simulink model "gm_HDL_pfc_gold_fi_og_vnl"  (R2024b)
settings: Solver=FixedStepDiscrete  StartTime=0.0  StopTime=.2  RelTol=1e-3
InitFcn:
  | fidelity_pfc_vals;
  | nbits=(2^12)-2;
  | load('C:\Users\Angel\Desktop\hil\pfc3ph\matlab\sim\sschdl\pfc_desktop\stateSpaceParameters.mat');
undefined symbols (not defined in the file or in its folder): a, b, c, DiscIntNeverNeededParam, fsw, Gs, s, stateSpaceParameters_1, t_ss, tsw
libraries: simulink x47, hdlmdlgenlib x24, hdlsllib x10, mcbcontrolslib x5, dspsrcs4 x3, slpidlib x2, hdlssclib x2, spsSVPWMGenerator2LevelLib x1, spsPLL3phLib x1, fillib x1
(part 3 of 5)

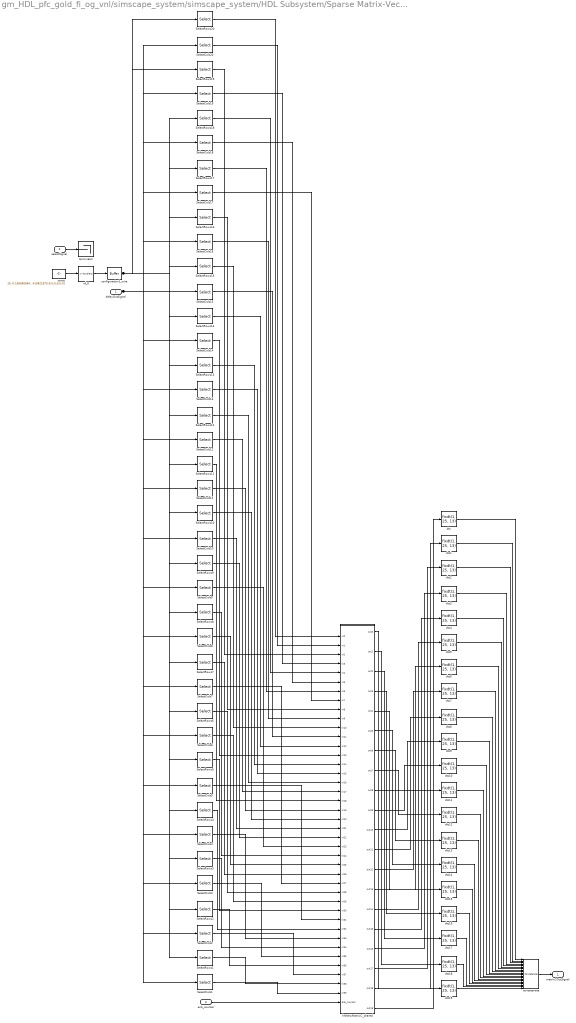
== system gm_HDL_pfc_gold_fi_og_vnl/simscape_system/simscape_system/HDL Subsystem/Sparse Matrix-Vector Product2 ==
  delayOutSignal : Inport  OutDataTypeStr=fixdt(1, 25, 13)  PortDimensions=[7]  SampleTime=1.38600138600139e-08
  selectSignal : Inport  Port=2  OutDataTypeStr=boolean  SampleTime=1.38600138600139e-08
  enb_counter : Inport  Port=3  OutDataTypeStr=fixdt(0, 6, 0)  SampleTime=1.38600138600139e-08
  SelectCols{1..20} (20 alike) : Selector  InputPortWidth=7  IndexOptions=Index vector (dialog)  Indices=double([1 2 3 4 5 6 7])  OutputSizes=double(1)
  SelectRows1 : Selector  InputPortWidth=140  IndexOptions=Index vector (dialog)  Indices=double([1 21 41 61 81 101 121])  OutputSizes=double(1)
  SelectRows10 : Selector  InputPortWidth=140  IndexOptions=Index vector (dialog)  Indices=double([10 30 50 70 90 110 130])  OutputSizes=double(1)
  SelectRows11 : Selector  InputPortWidth=140  IndexOptions=Index vector (dialog)  Indices=double([11 31 51 71 91 111 131])  OutputSizes=double(1)
  SelectRows12 : Selector  InputPortWidth=140  IndexOptions=Index vector (dialog)  Indices=double([12 32 52 72 92 112 132])  OutputSizes=double(1)
  SelectRows13 : Selector  InputPortWidth=140  IndexOptions=Index vector (dialog)  Indices=double([13 33 53 73 93 113 133])  OutputSizes=double(1)
  SelectRows14 : Selector  InputPortWidth=140  IndexOptions=Index vector (dialog)  Indices=double([14 34 54 74 94 114 134])  OutputSizes=double(1)
  SelectRows15 : Selector  InputPortWidth=140  IndexOptions=Index vector (dialog)  Indices=double([15 35 55 75 95 115 135])  OutputSizes=double(1)
  SelectRows16 : Selector  InputPortWidth=140  IndexOptions=Index vector (dialog)  Indices=double([16 36 56 76 96 116 136])  OutputSizes=double(1)
  SelectRows17 : Selector  InputPortWidth=140  IndexOptions=Index vector (dialog)  Indices=double([17 37 57 77 97 117 137])  OutputSizes=double(1)
  SelectRows18 : Selector  InputPortWidth=140  IndexOptions=Index vector (dialog)  Indices=double([18 38 58 78 98 118 138])  OutputSizes=double(1)
  SelectRows19 : Selector  InputPortWidth=140  IndexOptions=Index vector (dialog)  Indices=double([19 39 59 79 99 119 139])  OutputSizes=double(1)
  SelectRows2 : Selector  InputPortWidth=140  IndexOptions=Index vector (dialog)  Indices=double([2 22 42 62 82 102 122])  OutputSizes=double(1)
  SelectRows20 : Selector  InputPortWidth=140  IndexOptions=Index vector (dialog)  Indices=double([20 40 60 80 100 120 140])  OutputSizes=double(1)
  SelectRows3 : Selector  InputPortWidth=140  IndexOptions=Index vector (dialog)  Indices=double([3 23 43 63 83 103 123])  OutputSizes=double(1)
  SelectRows4 : Selector  InputPortWidth=140  IndexOptions=Index vector (dialog)  Indices=double([4 24 44 64 84 104 124])  OutputSizes=double(1)
  SelectRows5 : Selector  InputPortWidth=140  IndexOptions=Index vector (dialog)  Indices=double([5 25 45 65 85 105 125])  OutputSizes=double(1)
  SelectRows6 : Selector  InputPortWidth=140  IndexOptions=Index vector (dialog)  Indices=double([6 26 46 66 86 106 126])  OutputSizes=double(1)
  SelectRows7 : Selector  InputPortWidth=140  IndexOptions=Index vector (dialog)  Indices=double([7 27 47 67 87 107 127])  OutputSizes=double(1)
  SelectRows8 : Selector  InputPortWidth=140  IndexOptions=Index vector (dialog)  Indices=double([8 28 48 68 88 108 128])  OutputSizes=double(1)
  SelectRows9 : Selector  InputPortWidth=140  IndexOptions=Index vector (dialog)  Indices=double([9 29 49 69 89 109 129])  OutputSizes=double(1)
  concatenate : Concatenate  NumInputs=20
  configuration1_wire : hdlmdlgenlib/Buffer
  const : Constant  Value=[0;-0.16666698455810546875;-8.33333301544189453125;0.16666698455810546875;8.33333301544189453125;-0.08333301544189453125;-4.1666660308837890625;-0.08333301544189453125;-4.16666698455810546875;0.08333301544189453125;4.16666698455810546875;0.08333301544189453125;4.16666698455810546875;0;-0.16666698455810546875;-0.16666698455810546875;0.33333301544189453125;0;0;0;0;0.08333301544189453125;4.16666698455810546875;-0.08333301544189453125;-4.1666660308837890625;0.16666698455810546875;8.33333301544189453125;-0.08333301544189453125;-4.16666698455810546875;-0.16666698455810546875;-8.33333301544189453125;0.08333301544189453125;4.16666698455810546875;0;0.33333301544189453125;-0.16666698455810546875;-0.16666698455810546875;0;0;0;0;0.08333301544189453125;4.16666698455810546875;-0.08333301544189453125;-4.16666698455810546875;-0.08333301544189453125;-4.16666698455810546875;0.16666698455810546875;8.33333301544189453125;0.08333301544189453125;4.16666698455810546875;-0.16666698455810546875;-8.33333301544189453125;0;-0.16666698455810546875;0.33333301544189453125;-0.16666698455810546875;0;0;0;0;0.08333301544189453125;4.16666698455810546875;-0.08333301544189453125;-4.1666660308837890625;0.16666698455810546875;8.33333301544189453125;-0.08333301544189453125;-4.16666698455810546875;-0.16666698455810546875;-8.33333301544189453125;0.08333301544189453125;4.16666698455810546875;0;0.33333301544189453125;-0.16666698455810546875;-0.16666698455810546875;0;0;0;0;0.08333301544189453125;4.16666698455810546875;-0.08333301544189453125;-4.16666698455810546875;-0.08333301544189453125;-4.16666698455810546875;0.16666698455810546875;8.33333301544189453125;0.08333301544189453125;4.16666698455810546875;-0.16666698455810546875;-8.33333301544189453125;0;-0.16666698455810546875;0.33333301544189453125;-0.16666698455810546875;0;0;0;0;-0.16666698455810546875;-8.33333301544189453125;0.16666698455810546875;8.33333301544189453125;-0.08333301544189453125;-4.16666698455810546875;-0.08333301544189453125;-4.16666698455810546875;0.08333301544189453125;4.16666698455810546875;0.08333301544189453125;4.16666698455810546875;0;-0.16666698455810546875;-0.16666698455810546875;0.33333301544189453125;0;0;0;0;0.009998321533203125;0.4999103546142578125;0.009998321533203125;0.4999103546142578125;0.009998321533203125;0.4999103546142578125;0.009998321533203125;0.4999103546142578125;0.009998321533203125;0.4999103546142578125;0.009998321533203125;0.4999103546142578125;0.99981975555419921875;0;0;0;0;0;0]  OutDataTypeStr=fixdt(1, 25, 20)  SampleTime=1.38600138600139e-08
  dtc{,1..19} (20 alike) : DataTypeConversion  OutDataTypeStr=fixdt(1, 25, 13)  RndMeth=Nearest  SampleTime=1.38600138600139e-08  SaturateOnIntegerOverflow=off
  hNNewMatrixC_shared : Subsystem
  rd_0 : Delay  DelayLength=double(1)  InitialCondition=0  SampleTime=1.38600138600139e-08
  terminator : Terminator
  matrixCOutSignal : Outport  OutDataTypeStr=fixdt(1, 25, 13)  PortDimensions=[20]  SampleTime=1.38600138600139e-08
  wires:
  concatenate/1 -> matrixCOutSignal/1
  dtc19/1 -> concatenate/20
  dtc18/1 -> concatenate/19
  dtc17/1 -> concatenate/18
  dtc16/1 -> concatenate/17
  dtc14/1 -> concatenate/15
  dtc13/1 -> concatenate/14
  dtc12/1 -> concatenate/13
  dtc11/1 -> concatenate/12
  dtc10/1 -> concatenate/11
  dtc9/1 -> concatenate/10
  dtc8/1 -> concatenate/9
  dtc7/1 -> concatenate/8
  dtc6/1 -> concatenate/7
  dtc5/1 -> concatenate/6
  dtc4/1 -> concatenate/5
  dtc3/1 -> concatenate/4
  dtc1/1 -> concatenate/2
  dtc/1 -> concatenate/1
  hNNewMatrixC_shared/20(out19) -> dtc/1
  hNNewMatrixC_shared/19(out18) -> dtc1/1
  hNNewMatrixC_shared/18(out17) -> dtc2/1
  hNNewMatrixC_shared/16(out15) -> dtc4/1
  hNNewMatrixC_shared/13(out12) -> dtc7/1
  hNNewMatrixC_shared/12(out11) -> dtc8/1
  hNNewMatrixC_shared/9(out8) -> dtc11/1
  hNNewMatrixC_shared/1(out0) -> dtc19/1
  hNNewMatrixC_shared/10(out9) -> dtc10/1
  SelectCols1/1 -> hNNewMatrixC_shared/40(in39)
  hNNewMatrixC_shared/11(out10) -> dtc9/1
  SelectRows1/1 -> hNNewMatrixC_shared/39(in38)
  SelectCols2/1 -> hNNewMatrixC_shared/38(in37)
  SelectRows2/1 -> hNNewMatrixC_shared/37(in36)
  hNNewMatrixC_shared/6(out5) -> dtc14/1
  hNNewMatrixC_shared/7(out6) -> dtc13/1
  SelectRows3/1 -> hNNewMatrixC_shared/35(in34)
  hNNewMatrixC_shared/17(out16) -> dtc3/1
  SelectRows4/1 -> hNNewMatrixC_shared/33(in32)
  SelectCols5/1 -> hNNewMatrixC_shared/32(in31)
  SelectCols4/1 -> hNNewMatrixC_shared/34(in33)
  SelectCols6/1 -> hNNewMatrixC_shared/30(in29)
  SelectRows6/1 -> hNNewMatrixC_shared/29(in28)
  SelectCols7/1 -> hNNewMatrixC_shared/28(in27)
  SelectRows8/1 -> hNNewMatrixC_shared/25(in24)
  hNNewMatrixC_shared/5(out4) -> dtc15/1
  SelectCols9/1 -> hNNewMatrixC_shared/24(in23)
  SelectCols10/1 -> hNNewMatrixC_shared/22(in21)
  hNNewMatrixC_shared/2(out1) -> dtc18/1
  hNNewMatrixC_shared/3(out2) -> dtc17/1
  SelectRows10/1 -> hNNewMatrixC_shared/21(in20)
  SelectRows9/1 -> hNNewMatrixC_shared/23(in22)
  SelectCols11/1 -> hNNewMatrixC_shared/20(in19)
  SelectRows11/1 -> hNNewMatrixC_shared/19(in18)
  SelectCols8/1 -> hNNewMatrixC_shared/26(in25)
  SelectCols12/1 -> hNNewMatrixC_shared/18(in17)
  SelectRows5/1 -> hNNewMatrixC_shared/31(in30)
  hNNewMatrixC_shared/8(out7) -> dtc12/1
  SelectCols13/1 -> hNNewMatrixC_shared/16(in15)
  SelectRows14/1 -> hNNewMatrixC_shared/13(in12)
  SelectCols15/1 -> hNNewMatrixC_shared/12(in11)
  SelectRows15/1 -> hNNewMatrixC_shared/11(in10)
  SelectCols3/1 -> hNNewMatrixC_shared/36(in35)
  SelectCols17/1 -> hNNewMatrixC_shared/8(in7)
  enb_counter/1 -> hNNewMatrixC_shared/41(enb_counter)
  SelectCols16/1 -> hNNewMatrixC_shared/10(in9)
  hNNewMatrixC_shared/4(out3) -> dtc16/1
  SelectRows18/1 -> hNNewMatrixC_shared/5(in4)
  dtc2/1 -> concatenate/3
  SelectCols19/1 -> hNNewMatrixC_shared/4(in3)
  SelectRows19/1 -> hNNewMatrixC_shared/3(in2)
  SelectRows16/1 -> hNNewMatrixC_shared/9(in8)
  SelectCols14/1 -> hNNewMatrixC_shared/14(in13)
  SelectCols20/1 -> hNNewMatrixC_shared/2(in1)
  SelectRows20/1 -> hNNewMatrixC_shared/1(in0)
  delayOutSignal/1 -> SelectCols5/1, SelectCols1/1, SelectCols4/1, SelectCols2/1, SelectCols3/1, SelectCols6/1, SelectCols7/1, SelectCols20/1, SelectCols8/1, SelectCols9/1, SelectCols15/1, SelectCols10/1, SelectCols11/1, SelectCols12/1, SelectCols13/1, SelectCols14/1, SelectCols16/1, SelectCols17/1, SelectCols18/1, SelectCols19/1
  configuration1_wire/1 -> SelectRows20/1, SelectRows1/1, SelectRows4/1, SelectRows2/1, SelectRows15/1, SelectRows8/1, SelectRows3/1, SelectRows5/1, SelectRows7/1, SelectRows6/1, SelectRows9/1, SelectRows10/1, SelectRows11/1, SelectRows12/1, SelectRows13/1, SelectRows14/1, SelectRows16/1, SelectRows18/1, SelectRows17/1, SelectRows19/1
  SelectCols18/1 -> hNNewMatrixC_shared/6(in5)
  SelectRows12/1 -> hNNewMatrixC_shared/17(in16)
  const/1 -> rd_0/1
  SelectRows7/1 -> hNNewMatrixC_shared/27(in26)
  hNNewMatrixC_shared/14(out13) -> dtc6/1
  hNNewMatrixC_shared/15(out14) -> dtc5/1
  rd_0/1 -> configuration1_wire/1
  SelectRows17/1 -> hNNewMatrixC_shared/7(in6)
  dtc15/1 -> concatenate/16
  selectSignal/1 -> terminator/1
  SelectRows13/1 -> hNNewMatrixC_shared/15(in14)

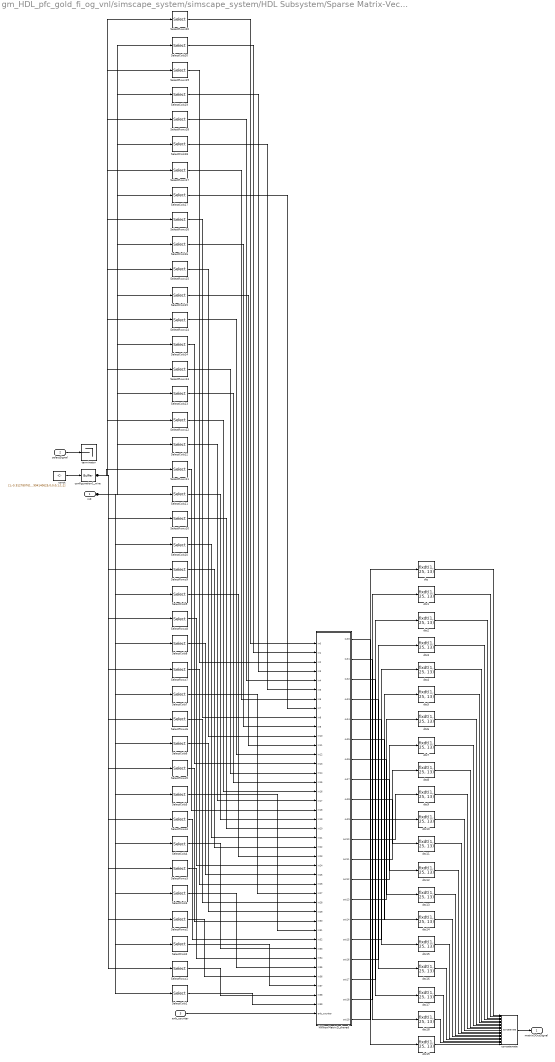
== system gm_HDL_pfc_gold_fi_og_vnl/simscape_system/simscape_system/HDL Subsystem/Sparse Matrix-Vector Product3 ==
  in0 : Inport  OutDataTypeStr=fixdt(1, 25, 13)  PortDimensions=[10]  SampleTime=1.38600138600139e-08
  selectSignal : Inport  Port=2  OutDataTypeStr=boolean  SampleTime=1.38600138600139e-08
  enb_counter : Inport  Port=3  OutDataTypeStr=fixdt(0, 6, 0)  SampleTime=1.38600138600139e-08
  SelectCols{1..17} (17 alike) : Selector  InputPortWidth=10  IndexOptions=Index vector (dialog)  Indices=double([1 2 3 4 5 6 7])  OutputSizes=double(1)
  SelectCols18 : Selector  InputPortWidth=10  IndexOptions=Index vector (dialog)  Indices=double([1 2 3 4 5 6 9])  OutputSizes=double(1)
  SelectCols19 : Selector  InputPortWidth=10  IndexOptions=Index vector (dialog)  Indices=double([1 2 3 4 5 6 10])  OutputSizes=double(1)
  SelectCols20 : Selector  InputPortWidth=10  IndexOptions=Index vector (dialog)  Indices=double([1 2 3 4 5 6 8])  OutputSizes=double(1)
  SelectRows1 : Selector  InputPortWidth=140  IndexOptions=Index vector (dialog)  Indices=double([1 21 41 61 81 101 121])  OutputSizes=double(1)
  SelectRows10 : Selector  InputPortWidth=140  IndexOptions=Index vector (dialog)  Indices=double([10 30 50 70 90 110 130])  OutputSizes=double(1)
  SelectRows11 : Selector  InputPortWidth=140  IndexOptions=Index vector (dialog)  Indices=double([11 31 51 71 91 111 131])  OutputSizes=double(1)
  SelectRows12 : Selector  InputPortWidth=140  IndexOptions=Index vector (dialog)  Indices=double([12 32 52 72 92 112 132])  OutputSizes=double(1)
  SelectRows13 : Selector  InputPortWidth=140  IndexOptions=Index vector (dialog)  Indices=double([13 33 53 73 93 113 133])  OutputSizes=double(1)
  SelectRows14 : Selector  InputPortWidth=140  IndexOptions=Index vector (dialog)  Indices=double([14 34 54 74 94 114 134])  OutputSizes=double(1)
  SelectRows15 : Selector  InputPortWidth=140  IndexOptions=Index vector (dialog)  Indices=double([15 35 55 75 95 115 135])  OutputSizes=double(1)
  SelectRows16 : Selector  InputPortWidth=140  IndexOptions=Index vector (dialog)  Indices=double([16 36 56 76 96 116 136])  OutputSizes=double(1)
  SelectRows17 : Selector  InputPortWidth=140  IndexOptions=Index vector (dialog)  Indices=double([17 37 57 77 97 117 137])  OutputSizes=double(1)
  SelectRows18 : Selector  InputPortWidth=140  IndexOptions=Index vector (dialog)  Indices=double([18 38 58 78 98 118 139])  OutputSizes=double(1)
  SelectRows19 : Selector  InputPortWidth=140  IndexOptions=Index vector (dialog)  Indices=double([19 39 59 79 99 119 140])  OutputSizes=double(1)
  SelectRows2 : Selector  InputPortWidth=140  IndexOptions=Index vector (dialog)  Indices=double([2 22 42 62 82 102 122])  OutputSizes=double(1)
  SelectRows20 : Selector  InputPortWidth=140  IndexOptions=Index vector (dialog)  Indices=double([20 40 60 80 100 120 138])  OutputSizes=double(1)
  SelectRows3 : Selector  InputPortWidth=140  IndexOptions=Index vector (dialog)  Indices=double([3 23 43 63 83 103 123])  OutputSizes=double(1)
  SelectRows4 : Selector  InputPortWidth=140  IndexOptions=Index vector (dialog)  Indices=double([4 24 44 64 84 104 124])  OutputSizes=double(1)
  SelectRows5 : Selector  InputPortWidth=140  IndexOptions=Index vector (dialog)  Indices=double([5 25 45 65 85 105 125])  OutputSizes=double(1)
  SelectRows6 : Selector  InputPortWidth=140  IndexOptions=Index vector (dialog)  Indices=double([6 26 46 66 86 106 126])  OutputSizes=double(1)
  SelectRows7 : Selector  InputPortWidth=140  IndexOptions=Index vector (dialog)  Indices=double([7 27 47 67 87 107 127])  OutputSizes=double(1)
  SelectRows8 : Selector  InputPortWidth=140  IndexOptions=Index vector (dialog)  Indices=double([8 28 48 68 88 108 128])  OutputSizes=double(1)
  SelectRows9 : Selector  InputPortWidth=140  IndexOptions=Index vector (dialog)  Indices=double([9 29 49 69 89 109 129])  OutputSizes=double(1)
  concatenate : Concatenate  NumInputs=20
  configuration1_wire : hdlmdlgenlib/Buffer
  const : Constant  Value=[1;-5.91278076171875e-05;-0.0030002593994140625;-5.91278076171875e-05;-0.0030002593994140625;-5.91278076171875e-05;-0.0030002593994140625;-5.91278076171875e-05;-0.0030002593994140625;-5.91278076171875e-05;-0.0030002593994140625;-5.91278076171875e-05;-0.0030002593994140625;-0.0059986114501953125;0;0;0;0;0;0;0;-0.499969482421875;25.001499176025390625;-0.499969482421875;-24.998500823974609375;3.0517578125e-05;0.001499176025390625;3.0517578125e-05;0.001499176025390625;3.0517578125e-05;0.001499176025390625;3.0517578125e-05;0.001499176025390625;0.0030002593994140625;0;0;0;0;0;0;0;-0.499969482421875;-24.998500823974609375;-0.499969482421875;25.001499176025390625;3.0517578125e-05;0.001499176025390625;3.0517578125e-05;0.001499176025390625;3.0517578125e-05;0.001499176025390625;3.0517578125e-05;0.001499176025390625;0.0030002593994140625;0;0;0;0;0;0;0;3.0517578125e-05;0.001499176025390625;3.0517578125e-05;0.001499176025390625;-0.499969482421875;25.001499176025390625;3.0517578125e-05;0.001499176025390625;-0.499969482421875;-24.998500823974609375;3.0517578125e-05;0.001499176025390625;0.0030002593994140625;0;0;0;0;0;0;0;3.0517578125e-05;0.001499176025390625;3.0517578125e-05;0.001499176025390625;3.0517578125e-05;0.001499176025390625;-0.499969482421875;25.001499176025390625;3.0517578125e-05;0.001499176025390625;-0.499969482421875;-24.998500823974609375;0.0030002593994140625;0;0;0;0;0;0;0;3.0517578125e-05;0.001499176025390625;3.0517578125e-05;0.001499176025390625;-0.499969482421875;-24.998500823974609375;3.0517578125e-05;0.001499176025390625;-0.499969482421875;25.001499176025390625;3.0517578125e-05;0.001499176025390625;0.0030002593994140625;0;0;0;0;0;0;0;3.0517578125e-05;0.001499176025390625;3.0517578125e-05;0.001499176025390625;3.0517578125e-05;0.001499176025390625;-0.499969482421875;-24.998500823974609375;3.0517578125e-05;0.001499176025390625;-0.499969482421875;25.001499176025390625;0.0030002593994140625;0;0;0;1;1;1]  OutDataTypeStr=fixdt(1, 25, 19)  SampleTime=1.38600138600139e-08
  dtc{,1..19} (20 alike) : DataTypeConversion  OutDataTypeStr=fixdt(1, 25, 13)  RndMeth=Nearest  SampleTime=1.38600138600139e-08  SaturateOnIntegerOverflow=off
  hNNewMatrixD_shared : Subsystem
  terminator : Terminator
  matrixDOutSignal : Outport  OutDataTypeStr=fixdt(1, 25, 13)  PortDimensions=[20]  SampleTime=1.38600138600139e-08
  wires:
  concatenate/1 -> matrixDOutSignal/1
  dtc19/1 -> concatenate/20
  dtc18/1 -> concatenate/19
  dtc17/1 -> concatenate/18
  dtc16/1 -> concatenate/17
  dtc15/1 -> concatenate/16
  dtc14/1 -> concatenate/15
  dtc13/1 -> concatenate/14
  dtc12/1 -> concatenate/13
  dtc11/1 -> concatenate/12
  dtc9/1 -> concatenate/10
  dtc8/1 -> concatenate/9
  dtc7/1 -> concatenate/8
  dtc4/1 -> concatenate/5
  dtc3/1 -> concatenate/4
  dtc2/1 -> concatenate/3
  dtc1/1 -> concatenate/2
  dtc/1 -> concatenate/1
  hNNewMatrixD_shared/20(out19) -> dtc/1
  hNNewMatrixD_shared/19(out18) -> dtc1/1
  dtc5/1 -> concatenate/6
  hNNewMatrixD_shared/15(out14) -> dtc5/1
  hNNewMatrixD_shared/10(out9) -> dtc10/1
  hNNewMatrixD_shared/7(out6) -> dtc13/1
  hNNewMatrixD_shared/4(out3) -> dtc16/1
  hNNewMatrixD_shared/6(out5) -> dtc14/1
  enb_counter/1 -> hNNewMatrixD_shared/41(enb_counter)
  hNNewMatrixD_shared/18(out17) -> dtc2/1
  SelectCols1/1 -> hNNewMatrixD_shared/40(in39)
  SelectRows1/1 -> hNNewMatrixD_shared/39(in38)
  SelectCols2/1 -> hNNewMatrixD_shared/38(in37)
  SelectRows2/1 -> hNNewMatrixD_shared/37(in36)
  SelectCols3/1 -> hNNewMatrixD_shared/36(in35)
  SelectRows3/1 -> hNNewMatrixD_shared/35(in34)
  hNNewMatrixD_shared/9(out8) -> dtc11/1
  SelectCols4/1 -> hNNewMatrixD_shared/34(in33)
  hNNewMatrixD_shared/8(out7) -> dtc12/1
  SelectCols5/1 -> hNNewMatrixD_shared/32(in31)
  SelectRows6/1 -> hNNewMatrixD_shared/29(in28)
  SelectCols7/1 -> hNNewMatrixD_shared/28(in27)
  hNNewMatrixD_shared/5(out4) -> dtc15/1
  SelectRows7/1 -> hNNewMatrixD_shared/27(in26)
  dtc10/1 -> concatenate/11
  SelectRows8/1 -> hNNewMatrixD_shared/25(in24)
  hNNewMatrixD_shared/11(out10) -> dtc9/1
  SelectCols10/1 -> hNNewMatrixD_shared/22(in21)
  SelectRows11/1 -> hNNewMatrixD_shared/19(in18)
  SelectRows12/1 -> hNNewMatrixD_shared/17(in16)
  SelectCols13/1 -> hNNewMatrixD_shared/16(in15)
  SelectCols11/1 -> hNNewMatrixD_shared/20(in19)
  SelectRows13/1 -> hNNewMatrixD_shared/15(in14)
  SelectCols14/1 -> hNNewMatrixD_shared/14(in13)
  SelectRows4/1 -> hNNewMatrixD_shared/33(in32)
  hNNewMatrixD_shared/2(out1) -> dtc18/1
  SelectRows14/1 -> hNNewMatrixD_shared/13(in12)
  hNNewMatrixD_shared/17(out16) -> dtc3/1
  SelectCols15/1 -> hNNewMatrixD_shared/12(in11)
  hNNewMatrixD_shared/12(out11) -> dtc8/1
  hNNewMatrixD_shared/16(out15) -> dtc4/1
  hNNewMatrixD_shared/14(out13) -> dtc6/1
  SelectRows15/1 -> hNNewMatrixD_shared/11(in10)
  SelectCols16/1 -> hNNewMatrixD_shared/10(in9)
  dtc6/1 -> concatenate/7
  hNNewMatrixD_shared/13(out12) -> dtc7/1
  SelectRows16/1 -> hNNewMatrixD_shared/9(in8)
  SelectCols17/1 -> hNNewMatrixD_shared/8(in7)
  SelectRows17/1 -> hNNewMatrixD_shared/7(in6)
  SelectCols18/1 -> hNNewMatrixD_shared/6(in5)
  SelectRows18/1 -> hNNewMatrixD_shared/5(in4)
  SelectCols9/1 -> hNNewMatrixD_shared/24(in23)
  hNNewMatrixD_shared/3(out2) -> dtc17/1
  SelectRows9/1 -> hNNewMatrixD_shared/23(in22)
  SelectRows19/1 -> hNNewMatrixD_shared/3(in2)
  SelectRows10/1 -> hNNewMatrixD_shared/21(in20)
  SelectRows20/1 -> hNNewMatrixD_shared/1(in0)
  SelectCols8/1 -> hNNewMatrixD_shared/26(in25)
  SelectCols6/1 -> hNNewMatrixD_shared/30(in29)
  in0/1 -> SelectCols5/1, SelectCols6/1, SelectCols1/1, SelectCols4/1, SelectCols10/1, SelectCols2/1, SelectCols9/1, SelectCols7/1, SelectCols3/1, SelectCols8/1, SelectCols11/1, SelectCols12/1, SelectCols13/1, SelectCols14/1, SelectCols15/1, SelectCols16/1, SelectCols17/1, SelectCols18/1, SelectCols19/1, SelectCols20/1
  configuration1_wire/1 -> SelectRows1/1, SelectRows7/1, SelectRows2/1, SelectRows5/1, SelectRows3/1, SelectRows17/1, SelectRows4/1, SelectRows6/1, SelectRows8/1, SelectRows9/1, SelectRows10/1, SelectRows11/1, SelectRows12/1, SelectRows13/1, SelectRows14/1, SelectRows15/1, SelectRows16/1, SelectRows18/1, SelectRows19/1, SelectRows20/1
  hNNewMatrixD_shared/1(out0) -> dtc19/1
  SelectCols20/1 -> hNNewMatrixD_shared/2(in1)
  SelectRows5/1 -> hNNewMatrixD_shared/31(in30)
  SelectCols19/1 -> hNNewMatrixD_shared/4(in3)
  const/1 -> configuration1_wire/1
  SelectCols12/1 -> hNNewMatrixD_shared/18(in17)
  selectSignal/1 -> terminator/1

== system gm_HDL_pfc_gold_fi_og_vnl/simscape_system/simscape_system/HDL Subsystem/streaming_partition_streamed ==
  in0 : Inport  OutDataTypeStr=fixdt(1, 25, 13)  PortDimensions=[7]  SampleTime=1.38600138600139e-08
  in1 : Inport  Port=2  OutDataTypeStr=fixdt(1, 25, 13)  PortDimensions=[7]  SampleTime=1.38600138600139e-08
  enb_counter : Inport  Port=3  OutDataTypeStr=fixdt(0, 6, 0)  SampleTime=1.38600138600139e-08
  Serializer_Subnetwork : Subsystem
  Serializer_Subnetwork1 : Subsystem
  counter : Subsystem
  delayInSignal_bypass : Subsystem
  dtc : hdlmdlgenlib/Buffer
  enb_counter_eq_20 : simulink/Logic and Bit Operations/Compare To Constant  relop===  const=double(20)  OutDataTypeStr=boolean
  enb_counter_ge_13 : simulink/Logic and Bit Operations/Compare To Constant  relop=>=  const=double(13)  OutDataTypeStr=boolean
  enb_counter_ge_13_and_enb_counter_le_19 : Logic  AllPortsSameDT=off  OutDataTypeStr=boolean  SampleTime=1.38600138600139e-08
  enb_counter_ge_14 : simulink/Logic and Bit Operations/Compare To Constant  relop=>=  const=double(14)  OutDataTypeStr=boolean
  enb_counter_ge_14_and_enb_counter_le_19 : Logic  AllPortsSameDT=off  OutDataTypeStr=boolean  SampleTime=1.38600138600139e-08
  enb_counter_le_19 : simulink/Logic and Bit Operations/Compare To Constant  relop=<=  const=double(19)  OutDataTypeStr=boolean
  enb_counter_le_191 : simulink/Logic and Bit Operations/Compare To Constant  relop=<=  const=double(19)  OutDataTypeStr=boolean
  rd_{0..4} (5 alike) : Delay  DelayLength=double(1)  InitialCondition=0  SampleTime=1.38600138600139e-08
  sumStateEqnComp : Sum  OutDataTypeStr=fixdt(1, 25, 13)  SampleTime=1.38600138600139e-08
  t : Mux  Inputs=2
  tappedDelay : Subsystem
  out0 : Outport  OutDataTypeStr=fixdt(1, 25, 13)  PortDimensions=[7]  SampleTime=1.38600138600139e-08
  wires:
  dtc/1 -> rd_3/1, tappedDelay/1(in0)
  sumStateEqnComp/1 -> dtc/1
  Serializer_Subnetwork/1(out0) -> sumStateEqnComp/1
  rd_1/1 -> Serializer_Subnetwork1/2(in1)
  in1/1 -> Serializer_Subnetwork1/1(in0)
  rd_2/1 -> t/1
  rd_0/1 -> Serializer_Subnetwork/2(in1)
  rd_3/1 -> delayInSignal_bypass/1(in0)
  in0/1 -> Serializer_Subnetwork/1(in0)
  rd_4/1 -> delayInSignal_bypass/2(in1)
  Serializer_Subnetwork1/1(out0) -> sumStateEqnComp/2
  tappedDelay/1(out0) -> rd_2/1
  counter/1(out0) -> rd_1/1, rd_0/1
  t/1 -> out0/1
  enb_counter_eq_20/1 -> rd_4/1
  enb_counter_le_191/1 -> enb_counter_ge_14_and_enb_counter_le_19/2
  enb_counter_ge_13_and_enb_counter_le_19/1 -> counter/Enable
  enb_counter_ge_14_and_enb_counter_le_19/1 -> tappedDelay/Enable
  enb_counter_le_19/1 -> enb_counter_ge_13_and_enb_counter_le_19/2
  enb_counter_ge_13/1 -> enb_counter_ge_13_and_enb_counter_le_19/1
  delayInSignal_bypass/1(out0) -> t/2
  enb_counter/1 -> enb_counter_le_191/1, enb_counter_le_19/1, enb_counter_ge_13/1, enb_counter_ge_14/1, enb_counter_eq_20/1
  enb_counter_ge_14/1 -> enb_counter_ge_14_and_enb_counter_le_19/1

== system gm_HDL_pfc_gold_fi_og_vnl/simscape_system/simscape_system/HDL Subsystem/streaming_partition_streamed1 ==
  in0 : Inport  OutDataTypeStr=fixdt(1, 25, 13)  PortDimensions=[7]  SampleTime=1.38600138600139e-08
  in1 : Inport  Port=2  OutDataTypeStr=boolean  SampleTime=1.38600138600139e-08
  in2 : Inport  Port=3  OutDataTypeStr=fixdt(1, 25, 13)  PortDimensions=[7]  SampleTime=1.38600138600139e-08
  enb_counter : Inport  Port=4  OutDataTypeStr=fixdt(0, 6, 0)  SampleTime=1.38600138600139e-08
  Serializer_Subnetwork : Subsystem
  Serializer_Subnetwork1 : Subsystem
  State_switch : Switch  Criteria=u2 ~= 0  Threshold=double(0)  OutDataTypeStr=fixdt(1, 25, 13)  SampleTime=1.38600138600139e-08  SaturateOnIntegerOverflow=off  InputSameDT=off
  counter : Subsystem
  delayOutSignal_bypass : Subsystem
  enb_counter_eq_6 : simulink/Logic and Bit Operations/Compare To Constant  relop===  const=double(6)  OutDataTypeStr=boolean
  enb_counter_le_5 : simulink/Logic and Bit Operations/Compare To Constant  relop=<=  const=double(5)  OutDataTypeStr=boolean
  enb_counter_le_6 : simulink/Logic and Bit Operations/Compare To Constant  relop=<=  const=double(6)  OutDataTypeStr=boolean
  t : Mux  Inputs=2
  tappedDelay : Subsystem
  out0 : Outport  OutDataTypeStr=fixdt(1, 25, 13)  PortDimensions=[7]  SampleTime=1.38600138600139e-08
  wires:
  delayOutSignal_bypass/1(out0) -> t/2
  enb_counter_eq_6/1 -> delayOutSignal_bypass/2(in1)
  State_switch/1 -> delayOutSignal_bypass/1(in0), tappedDelay/1(in0)
  Serializer_Subnetwork1/1(out0) -> State_switch/3
  in2/1 -> Serializer_Subnetwork1/1(in0)
  counter/1(out0) -> Serializer_Subnetwork/2(in1), Serializer_Subnetwork1/2(in1)
  t/1 -> out0/1
  Serializer_Subnetwork/1(out0) -> State_switch/1
  in0/1 -> Serializer_Subnetwork/1(in0)
  tappedDelay/1(out0) -> t/1
  enb_counter_le_5/1 -> tappedDelay/Enable
  enb_counter_le_6/1 -> counter/Enable
  in1/1 -> State_switch/2
  enb_counter/1 -> enb_counter_eq_6/1, enb_counter_le_5/1, enb_counter_le_6/1

== system gm_HDL_pfc_gold_fi_og_vnl/simscape_system_vnl/HDL Subsystem/HDL Algorithm/Output ==
  In1 : Inport
  State : Inport  Port=2
  Sel : Inport  Port=3  LockScale=on
  Bias : Terminator
  Mux : Mux  Inputs=2
  Output Update : hdlssclib/NFPSparseConstMultiply  MatrixSource=Dialog  constMatrix=single([stateSpaceParameters_1.Cd stateSpaceParameters_1.Dd])  MatrixType=single  MatrixSize=[1 1]  ColumnIndices=[1]  RowIndices=[1]  PropDataType=single  defWL=48
  Out1 : Outport  VectorParamsAs1DForOutWhenUnconnected=off
  wires:
  Output Update/1 -> Out1/1
  Sel/1 -> Output Update/2, Bias/1
  In1/1 -> Mux/2
  Mux/1 -> Output Update/1
  State/1 -> Mux/1

== system gm_HDL_pfc_gold_fi_og_vnl/simscape_system_vnl/HDL Subsystem/HDL Algorithm/State Update ==
  In1 : Inport
  State : Inport  Port=2
  Sel : Inport  Port=3  LockScale=on
  Bias : Terminator
  Mux : Mux  Inputs=2
  State Update : hdlssclib/NFPSparseConstMultiply  MatrixSource=Dialog  constMatrix=single([stateSpaceParameters_1.Ad stateSpaceParameters_1.Bd])  MatrixType=single  MatrixSize=[1 1]  ColumnIndices=[1]  RowIndices=[1]  PropDataType=single  defWL=43
  State Out : Outport  VectorParamsAs1DForOutWhenUnconnected=off
  wires:
  State Update/1 -> State Out/1
  Sel/1 -> State Update/2, Bias/1
  Mux/1 -> State Update/1
  In1/1 -> Mux/2
  State/1 -> Mux/1

== system gm_HDL_pfc_gold_fi_og_vnl/simscape_system/simscape_system/FET_CTRL/crp_temp_streamed/Discrete-Time Integrator_u_sat_bypass ==
  in0 : Inport  OutDataTypeStr=fixdt(1, 18, 8)  PortDimensions=[5]  SampleTime=1.38600138600139e-08
  in1 : Inport  Port=2  OutDataTypeStr=boolean  SampleTime=1.38600138600139e-08
  Discrete-Time Integrator_u_sat_enb : Switch  Criteria=u2 ~= 0  Threshold=double(0)  OutDataTypeStr=fixdt(1, 18, 8)  SampleTime=1.38600138600139e-08  SaturateOnIntegerOverflow=off  InputSameDT=off
  Discrete-Time Integrator_u_sat_state : Delay  DelayLength=double(1)  InitialCondition=0  SampleTime=1.38600138600139e-08
  out0 : Outport  OutDataTypeStr=fixdt(1, 18, 8)  PortDimensions=[5]  SampleTime=1.38600138600139e-08
  wires:
  Discrete-Time Integrator_u_sat_enb/1 -> out0/1, Discrete-Time Integrator_u_sat_state/1
  in1/1 -> Discrete-Time Integrator_u_sat_enb/2
  Discrete-Time Integrator_u_sat_state/1 -> Discrete-Time Integrator_u_sat_enb/3
  in0/1 -> Discrete-Time Integrator_u_sat_enb/1

== system gm_HDL_pfc_gold_fi_og_vnl/simscape_system/simscape_system/FET_CTRL/crp_temp_streamed/Discrete-Time Integrator_u_sat_bypass1 ==
  in0 : Inport  OutDataTypeStr=fixdt(1, 18, 8)  SampleTime=1.38600138600139e-08
  in1 : Inport  Port=2  OutDataTypeStr=boolean  SampleTime=1.38600138600139e-08
  Discrete-Time Integrator_u_sat_enb : Switch  Criteria=u2 ~= 0  Threshold=double(0)  OutDataTypeStr=fixdt(1, 18, 8)  SampleTime=1.38600138600139e-08  SaturateOnIntegerOverflow=off  InputSameDT=off
  Discrete-Time Integrator_u_sat_state : Delay  DelayLength=double(1)  InitialCondition=0  SampleTime=1.38600138600139e-08
  out0 : Outport  OutDataTypeStr=fixdt(1, 18, 8)  SampleTime=1.38600138600139e-08
  wires:
  Discrete-Time Integrator_u_sat_enb/1 -> out0/1, Discrete-Time Integrator_u_sat_state/1
  in1/1 -> Discrete-Time Integrator_u_sat_enb/2
  Discrete-Time Integrator_u_sat_state/1 -> Discrete-Time Integrator_u_sat_enb/3
  in0/1 -> Discrete-Time Integrator_u_sat_enb/1

== system gm_HDL_pfc_gold_fi_og_vnl/simscape_system/simscape_system/FET_CTRL/crp_temp_streamed/Serializer_Subnetwork ==
  in0 : Inport  OutDataTypeStr=fixdt(1, 18, 8)  PortDimensions=[6]  SampleTime=1.38600138600139e-08
  in1 : Inport  Port=2  OutDataTypeStr=fixdt(0, 3, 0)  SampleTime=1.38600138600139e-08
  ratechange_splitcomp : Demux  Outputs=6
  splitcomp_multiport : MultiPortSwitch  DataPortOrder=Zero-based contiguous  Inputs=6  DiagnosticForDefault=None  zeroidx=on  OutDataTypeStr=fixdt(1, 18, 8)  SampleTime=1.38600138600139e-08  SaturateOnIntegerOverflow=off  InputSameDT=off
  out0 : Outport  OutDataTypeStr=fixdt(1, 18, 8)  SampleTime=1.38600138600139e-08
  wires:
  splitcomp_multiport/1 -> out0/1
  ratechange_splitcomp/6 -> splitcomp_multiport/7
  ratechange_splitcomp/5 -> splitcomp_multiport/6
  ratechange_splitcomp/4 -> splitcomp_multiport/5
  ratechange_splitcomp/3 -> splitcomp_multiport/4
  ratechange_splitcomp/2 -> splitcomp_multiport/3
  ratechange_splitcomp/1 -> splitcomp_multiport/2
  in1/1 -> splitcomp_multiport/1
  in0/1 -> ratechange_splitcomp/1

== system gm_HDL_pfc_gold_fi_og_vnl/simscape_system/simscape_system/FET_CTRL/crp_temp_streamed/Serializer_Subnetwork1 ==
  in0 : Inport  OutDataTypeStr=boolean  PortDimensions=[6]  SampleTime=1.38600138600139e-08
  in1 : Inport  Port=2  OutDataTypeStr=fixdt(0, 3, 0)  SampleTime=1.38600138600139e-08
  ratechange_splitcomp : Demux  Outputs=6
  splitcomp_multiport : MultiPortSwitch  DataPortOrder=Zero-based contiguous  Inputs=6  DiagnosticForDefault=None  zeroidx=on  SampleTime=1.38600138600139e-08  SaturateOnIntegerOverflow=off  InputSameDT=off
  out0 : Outport  OutDataTypeStr=boolean  SampleTime=1.38600138600139e-08
  wires:
  ratechange_splitcomp/6 -> splitcomp_multiport/7
  ratechange_splitcomp/5 -> splitcomp_multiport/6
  ratechange_splitcomp/3 -> splitcomp_multiport/4
  ratechange_splitcomp/2 -> splitcomp_multiport/3
  splitcomp_multiport/1 -> out0/1
  ratechange_splitcomp/4 -> splitcomp_multiport/5
  ratechange_splitcomp/1 -> splitcomp_multiport/2
  in1/1 -> splitcomp_multiport/1
  in0/1 -> ratechange_splitcomp/1

== system gm_HDL_pfc_gold_fi_og_vnl/simscape_system/simscape_system/FET_CTRL/crp_temp_streamed/Serializer_Subnetwork2 ==
  in0 : Inport  OutDataTypeStr=fixdt(1, 18, 6)  PortDimensions=[6]  SampleTime=1.38600138600139e-08
  in1 : Inport  Port=2  OutDataTypeStr=fixdt(0, 3, 0)  SampleTime=1.38600138600139e-08
  ratechange_splitcomp : Demux  Outputs=6
  splitcomp_multiport : MultiPortSwitch  DataPortOrder=Zero-based contiguous  Inputs=6  DiagnosticForDefault=None  zeroidx=on  OutDataTypeStr=fixdt(1, 18, 6)  SampleTime=1.38600138600139e-08  SaturateOnIntegerOverflow=off  InputSameDT=off
  out0 : Outport  OutDataTypeStr=fixdt(1, 18, 6)  SampleTime=1.38600138600139e-08
  wires:
  splitcomp_multiport/1 -> out0/1
  ratechange_splitcomp/6 -> splitcomp_multiport/7
  ratechange_splitcomp/5 -> splitcomp_multiport/6
  ratechange_splitcomp/4 -> splitcomp_multiport/5
  in1/1 -> splitcomp_multiport/1
  ratechange_splitcomp/3 -> splitcomp_multiport/4
  ratechange_splitcomp/2 -> splitcomp_multiport/3
  ratechange_splitcomp/1 -> splitcomp_multiport/2
  in0/1 -> ratechange_splitcomp/1

== system gm_HDL_pfc_gold_fi_og_vnl/simscape_system/simscape_system/FET_CTRL/crp_temp_streamed/Serializer_Subnetwork3 ==
  in0 : Inport  OutDataTypeStr=fixdt(1, 18, 6)  PortDimensions=[6]  SampleTime=1.38600138600139e-08
  in1 : Inport  Port=2  OutDataTypeStr=fixdt(0, 3, 0)  SampleTime=1.38600138600139e-08
  ratechange_splitcomp : Demux  Outputs=6
  splitcomp_multiport : MultiPortSwitch  DataPortOrder=Zero-based contiguous  Inputs=6  DiagnosticForDefault=None  zeroidx=on  OutDataTypeStr=fixdt(1, 18, 6)  SampleTime=1.38600138600139e-08  SaturateOnIntegerOverflow=off  InputSameDT=off
  out0 : Outport  OutDataTypeStr=fixdt(1, 18, 6)  SampleTime=1.38600138600139e-08
  wires:
  splitcomp_multiport/1 -> out0/1
  ratechange_splitcomp/6 -> splitcomp_multiport/7
  ratechange_splitcomp/5 -> splitcomp_multiport/6
  ratechange_splitcomp/4 -> splitcomp_multiport/5
  ratechange_splitcomp/1 -> splitcomp_multiport/2
  in1/1 -> splitcomp_multiport/1
  in0/1 -> ratechange_splitcomp/1
  ratechange_splitcomp/3 -> splitcomp_multiport/4
  ratechange_splitcomp/2 -> splitcomp_multiport/3

== system gm_HDL_pfc_gold_fi_og_vnl/simscape_system/simscape_system/FET_CTRL/crp_temp_streamed/buffSig_bypass ==
  in0 : Inport  OutDataTypeStr=fixdt(1, 18, 8)  PortDimensions=[5]  SampleTime=1.38600138600139e-08
  in1 : Inport  Port=2  OutDataTypeStr=boolean  SampleTime=1.38600138600139e-08
  buffSig_enb : Switch  Criteria=u2 ~= 0  Threshold=double(0)  OutDataTypeStr=fixdt(1, 18, 8)  SampleTime=1.38600138600139e-08  SaturateOnIntegerOverflow=off  InputSameDT=off
  buffSig_state : Delay  DelayLength=double(1)  InitialCondition=0  SampleTime=1.38600138600139e-08
  out0 : Outport  OutDataTypeStr=fixdt(1, 18, 8)  PortDimensions=[5]  SampleTime=1.38600138600139e-08
  wires:
  buffSig_enb/1 -> out0/1, buffSig_state/1
  in1/1 -> buffSig_enb/2
  in0/1 -> buffSig_enb/1
  buffSig_state/1 -> buffSig_enb/3

== system gm_HDL_pfc_gold_fi_og_vnl/simscape_system/simscape_system/FET_CTRL/crp_temp_streamed/buffSig_bypass1 ==
  in0 : Inport  OutDataTypeStr=fixdt(1, 18, 8)  SampleTime=1.38600138600139e-08
  in1 : Inport  Port=2  OutDataTypeStr=boolean  SampleTime=1.38600138600139e-08
  buffSig_enb : Switch  Criteria=u2 ~= 0  Threshold=double(0)  OutDataTypeStr=fixdt(1, 18, 8)  SampleTime=1.38600138600139e-08  SaturateOnIntegerOverflow=off  InputSameDT=off
  buffSig_state : Delay  DelayLength=double(1)  InitialCondition=0  SampleTime=1.38600138600139e-08
  out0 : Outport  OutDataTypeStr=fixdt(1, 18, 8)  SampleTime=1.38600138600139e-08
  wires:
  buffSig_enb/1 -> out0/1, buffSig_state/1
  buffSig_state/1 -> buffSig_enb/3
  in1/1 -> buffSig_enb/2
  in0/1 -> buffSig_enb/1

== system gm_HDL_pfc_gold_fi_og_vnl/simscape_system/simscape_system/FET_CTRL/crp_temp_streamed/counter ==
  globalSchedule : EnablePort  OutDataTypeStr=boolean
  ctr_0_5 : hdlsllib/Sources/HDL Counter  CountType=Count limited  CountInit=double(0)  CountStep=double(1)  CountMax=double(5)  CountFromType=Initial value  CountFrom=double(0)  CountResetPort=off  CountLoadPort=off  CountEnbPort=off  CountDirPort=off  CountHitOutputPort=off  CountDataType=Unsigned  CountWordLen=3  CountFracLen=0  CountSampTime=1.38600138600139e-08
  out0 : Outport  OutDataTypeStr=fixdt(0, 3, 0)  SampleTime=1.38600138600139e-08  InitialOutput=0
  wires:
  ctr_0_5/1 -> out0/1

== system gm_HDL_pfc_gold_fi_og_vnl/simscape_system/simscape_system/FET_CTRL/crp_temp_streamed/tappedDelay ==
  in0 : Inport  OutDataTypeStr=fixdt(1, 18, 8)  SampleTime=1.38600138600139e-08
  globalSchedule : EnablePort  OutDataTypeStr=boolean
  StateControl : StateControl  StateControl=Synchronous
  tapped_delay : simulink/Discrete/Tapped Delay  vinit=0  samptime=-1  NumDelays=double(5)  DelayOrder=Oldest  includeCurrent=off
  out0 : Outport  OutDataTypeStr=fixdt(1, 18, 8)  PortDimensions=[5]  SampleTime=1.38600138600139e-08  InitialOutput=0
  wires:
  tapped_delay/1 -> out0/1
  in0/1 -> tapped_delay/1

== system gm_HDL_pfc_gold_fi_og_vnl/simscape_system/simscape_system/FET_CTRL/crp_temp_streamed/tappedDelay1 ==
  in0 : Inport  OutDataTypeStr=fixdt(1, 18, 8)  SampleTime=1.38600138600139e-08
  globalSchedule : EnablePort  OutDataTypeStr=boolean
  StateControl : StateControl  StateControl=Synchronous
  tapped_delay : simulink/Discrete/Tapped Delay  vinit=0  samptime=-1  NumDelays=double(5)  DelayOrder=Oldest  includeCurrent=off
  out0 : Outport  OutDataTypeStr=fixdt(1, 18, 8)  PortDimensions=[5]  SampleTime=1.38600138600139e-08  InitialOutput=0
  wires:
  tapped_delay/1 -> out0/1
  in0/1 -> tapped_delay/1

== system gm_HDL_pfc_gold_fi_og_vnl/simscape_system/simscape_system/HDL Subsystem/Sparse Matrix-Vector Product/hNNewMatrixB_shared ==
  in0 : Inport  OutDataTypeStr=fixdt(1, 25, 31)  PortDimensions=[9]  SampleTime=1.38600138600139e-08
  in1 : Inport  Port=2  OutDataTypeStr=fixdt(1, 25, 13)  PortDimensions=[9]  SampleTime=1.38600138600139e-08
  in2 : Inport  Port=3  OutDataTypeStr=fixdt(1, 25, 31)  PortDimensions=[9]  SampleTime=1.38600138600139e-08
  in3 : Inport  Port=4  OutDataTypeStr=fixdt(1, 25, 13)  PortDimensions=[9]  SampleTime=1.38600138600139e-08
  in4 : Inport  Port=5  OutDataTypeStr=fixdt(1, 25, 31)  PortDimensions=[9]  SampleTime=1.38600138600139e-08
  in5 : Inport  Port=6  OutDataTypeStr=fixdt(1, 25, 13)  PortDimensions=[9]  SampleTime=1.38600138600139e-08
  in6 : Inport  Port=7  OutDataTypeStr=fixdt(1, 25, 31)  PortDimensions=[9]  SampleTime=1.38600138600139e-08
  in7 : Inport  Port=8  OutDataTypeStr=fixdt(1, 25, 13)  PortDimensions=[9]  SampleTime=1.38600138600139e-08
  in8 : Inport  Port=9  OutDataTypeStr=fixdt(1, 25, 31)  PortDimensions=[9]  SampleTime=1.38600138600139e-08
  in9 : Inport  Port=10  OutDataTypeStr=fixdt(1, 25, 13)  PortDimensions=[9]  SampleTime=1.38600138600139e-08
  in10 : Inport  Port=11  OutDataTypeStr=fixdt(1, 25, 31)  PortDimensions=[9]  SampleTime=1.38600138600139e-08
  in11 : Inport  Port=12  OutDataTypeStr=fixdt(1, 25, 13)  PortDimensions=[9]  SampleTime=1.38600138600139e-08
  in12 : Inport  Port=13  OutDataTypeStr=fixdt(1, 25, 31)  PortDimensions=[9]  SampleTime=1.38600138600139e-08
  in13 : Inport  Port=14  OutDataTypeStr=fixdt(1, 25, 13)  PortDimensions=[9]  SampleTime=1.38600138600139e-08
  enb_counter : Inport  Port=15  OutDataTypeStr=fixdt(0, 6, 0)  SampleTime=1.38600138600139e-08
  Serializer_Subnetwork : Subsystem
  Serializer_Subnetwork1 : Subsystem
  counter : Subsystem
  demux : Demux  Outputs=6
  dot_product1_bypass : Subsystem
  dot_product_9 : Subsystem
  enb_counter_eq_13 : simulink/Logic and Bit Operations/Compare To Constant  relop===  const=double(13)  OutDataTypeStr=boolean
  enb_counter_ge_7 : simulink/Logic and Bit Operations/Compare To Constant  relop=>=  const=double(7)  OutDataTypeStr=boolean
  enb_counter_ge_7_and_enb_counter_le_12 : Logic  AllPortsSameDT=off  OutDataTypeStr=boolean  SampleTime=1.38600138600139e-08
  enb_counter_le_12 : simulink/Logic and Bit Operations/Compare To Constant  relop=<=  const=double(12)  OutDataTypeStr=boolean
  enb_counter_le_6 : simulink/Logic and Bit Operations/Compare To Constant  relop=<=  const=double(6)  OutDataTypeStr=boolean
  mux : Mux  Inputs=7
  mux1 : Mux  Inputs=7
  rd_0 : Delay  DelayLength=double(5)  InitialCondition=0  SampleTime=1.38600138600139e-08
  tappedDelay : Subsystem
  out0 : Outport  OutDataTypeStr=fixdt(1, 50, 44)  SampleTime=1.38600138600139e-08
  out1 : Outport  Port=2  OutDataTypeStr=fixdt(1, 50, 44)  SampleTime=1.38600138600139e-08
  out2 : Outport  Port=3  OutDataTypeStr=fixdt(1, 50, 44)  SampleTime=1.38600138600139e-08
  out3 : Outport  Port=4  OutDataTypeStr=fixdt(1, 50, 44)  SampleTime=1.38600138600139e-08
  out4 : Outport  Port=5  OutDataTypeStr=fixdt(1, 50, 44)  SampleTime=1.38600138600139e-08
  out5 : Outport  Port=6  OutDataTypeStr=fixdt(1, 50, 44)  SampleTime=1.38600138600139e-08
  out6 : Outport  Port=7  OutDataTypeStr=fixdt(1, 50, 44)  SampleTime=1.38600138600139e-08
  wires:
  demux/4 -> out3/1
  demux/5 -> out4/1
  demux/6 -> out5/1
  demux/1 -> out0/1
  demux/2 -> out1/1
  demux/3 -> out2/1
  tappedDelay/1(out0) -> demux/1
  dot_product1_bypass/1(out0) -> out6/1
  dot_product_9/1(out1) -> dot_product1_bypass/1(in0), tappedDelay/1(in0)
  Serializer_Subnetwork1/1(out0) -> dot_product_9/2(in2)
  rd_0/1 -> Serializer_Subnetwork1/2(in1)
  mux1/1 -> Serializer_Subnetwork1/1(in0)
  Serializer_Subnetwork/1(out0) -> dot_product_9/1(in1)
  enb_counter_ge_7_and_enb_counter_le_12/1 -> tappedDelay/Enable
  in11/1 -> mux1/6
  in9/1 -> mux1/5
  in7/1 -> mux1/4
  enb_counter_eq_13/1 -> dot_product1_bypass/2(in1)
  counter/1(out0) -> Serializer_Subnetwork/2(in1), rd_0/1
  in5/1 -> mux1/3
  in3/1 -> mux1/2
  in1/1 -> mux1/1
  mux/1 -> Serializer_Subnetwork/1(in0)
  enb_counter_le_12/1 -> enb_counter_ge_7_and_enb_counter_le_12/2
  enb_counter_ge_7/1 -> enb_counter_ge_7_and_enb_counter_le_12/1
  enb_counter_le_6/1 -> counter/Enable
  in10/1 -> mux/6
  in8/1 -> mux/5
  in6/1 -> mux/4
  in12/1 -> mux/7
  in13/1 -> mux1/7
  in4/1 -> mux/3
  in2/1 -> mux/2
  in0/1 -> mux/1
  enb_counter/1 -> enb_counter_ge_7/1, enb_counter_le_6/1, enb_counter_eq_13/1, enb_counter_le_12/1

== system gm_HDL_pfc_gold_fi_og_vnl/simscape_system/simscape_system/HDL Subsystem/Sparse Matrix-Vector Product1/hNNewMatrixA_shared ==
  in0 : Inport  OutDataTypeStr=fixdt(1, 25, 24)  PortDimensions=[6]  SampleTime=1.38600138600139e-08
  in1 : Inport  Port=2  OutDataTypeStr=fixdt(1, 25, 13)  PortDimensions=[6]  SampleTime=1.38600138600139e-08
  in2 : Inport  Port=3  OutDataTypeStr=fixdt(1, 25, 24)  PortDimensions=[6]  SampleTime=1.38600138600139e-08
  in3 : Inport  Port=4  OutDataTypeStr=fixdt(1, 25, 13)  PortDimensions=[6]  SampleTime=1.38600138600139e-08
  in4 : Inport  Port=5  OutDataTypeStr=fixdt(1, 25, 24)  PortDimensions=[6]  SampleTime=1.38600138600139e-08
  in5 : Inport  Port=6  OutDataTypeStr=fixdt(1, 25, 13)  PortDimensions=[6]  SampleTime=1.38600138600139e-08
  in6 : Inport  Port=7  OutDataTypeStr=fixdt(1, 25, 24)  PortDimensions=[6]  SampleTime=1.38600138600139e-08
  in7 : Inport  Port=8  OutDataTypeStr=fixdt(1, 25, 13)  PortDimensions=[6]  SampleTime=1.38600138600139e-08
  in8 : Inport  Port=9  OutDataTypeStr=fixdt(1, 25, 24)  PortDimensions=[6]  SampleTime=1.38600138600139e-08
  in9 : Inport  Port=10  OutDataTypeStr=fixdt(1, 25, 13)  PortDimensions=[6]  SampleTime=1.38600138600139e-08
  in10 : Inport  Port=11  OutDataTypeStr=fixdt(1, 25, 24)  PortDimensions=[6]  SampleTime=1.38600138600139e-08
  in11 : Inport  Port=12  OutDataTypeStr=fixdt(1, 25, 13)  PortDimensions=[6]  SampleTime=1.38600138600139e-08
  in12 : Inport  Port=13  OutDataTypeStr=fixdt(1, 25, 24)  PortDimensions=[6]  SampleTime=1.38600138600139e-08
  in13 : Inport  Port=14  OutDataTypeStr=fixdt(1, 25, 13)  PortDimensions=[6]  SampleTime=1.38600138600139e-08
  enb_counter : Inport  Port=15  OutDataTypeStr=fixdt(0, 6, 0)  SampleTime=1.38600138600139e-08
  Serializer_Subnetwork : Subsystem
  Serializer_Subnetwork1 : Subsystem
  counter : Subsystem
  demux : Demux  Outputs=6
  dot_product1_bypass : Subsystem
  dot_product_6 : Subsystem
  enb_counter_eq_14 : simulink/Logic and Bit Operations/Compare To Constant  relop===  const=double(14)  OutDataTypeStr=boolean
  enb_counter_ge_8 : simulink/Logic and Bit Operations/Compare To Constant  relop=>=  const=double(8)  OutDataTypeStr=boolean
  enb_counter_ge_8_and_enb_counter_le_13 : Logic  AllPortsSameDT=off  OutDataTypeStr=boolean  SampleTime=1.38600138600139e-08
  enb_counter_le_13 : simulink/Logic and Bit Operations/Compare To Constant  relop=<=  const=double(13)  OutDataTypeStr=boolean
  enb_counter_le_6 : simulink/Logic and Bit Operations/Compare To Constant  relop=<=  const=double(6)  OutDataTypeStr=boolean
  mux : Mux  Inputs=7
  mux1 : Mux  Inputs=7
  rd_0 : Delay  DelayLength=double(6)  InitialCondition=0  SampleTime=1.38600138600139e-08
  tappedDelay : Subsystem
  out0 : Outport  OutDataTypeStr=fixdt(1, 50, 37)  SampleTime=1.38600138600139e-08
  out1 : Outport  Port=2  OutDataTypeStr=fixdt(1, 50, 37)  SampleTime=1.38600138600139e-08
  out2 : Outport  Port=3  OutDataTypeStr=fixdt(1, 50, 37)  SampleTime=1.38600138600139e-08
  out3 : Outport  Port=4  OutDataTypeStr=fixdt(1, 50, 37)  SampleTime=1.38600138600139e-08
  out4 : Outport  Port=5  OutDataTypeStr=fixdt(1, 50, 37)  SampleTime=1.38600138600139e-08
  out5 : Outport  Port=6  OutDataTypeStr=fixdt(1, 50, 37)  SampleTime=1.38600138600139e-08
  out6 : Outport  Port=7  OutDataTypeStr=fixdt(1, 50, 37)  SampleTime=1.38600138600139e-08
  wires:
  demux/2 -> out1/1
  demux/1 -> out0/1
  tappedDelay/1(out0) -> demux/1
  dot_product_6/1(out1) -> dot_product1_bypass/1(in0), tappedDelay/1(in0)
  enb_counter_eq_14/1 -> dot_product1_bypass/2(in1)
  rd_0/1 -> Serializer_Subnetwork1/2(in1)
  mux1/1 -> Serializer_Subnetwork1/1(in0)
  Serializer_Subnetwork/1(out0) -> dot_product_6/1(in1)
  enb_counter_ge_8_and_enb_counter_le_13/1 -> tappedDelay/Enable
  in13/1 -> mux1/7
  demux/6 -> out5/1
  in11/1 -> mux1/6
  dot_product1_bypass/1(out0) -> out6/1
  demux/3 -> out2/1
  demux/4 -> out3/1
  demux/5 -> out4/1
  in7/1 -> mux1/4
  counter/1(out0) -> Serializer_Subnetwork/2(in1), rd_0/1
  in3/1 -> mux1/2
  Serializer_Subnetwork1/1(out0) -> dot_product_6/2(in2)
  enb_counter_le_13/1 -> enb_counter_ge_8_and_enb_counter_le_13/2
  mux/1 -> Serializer_Subnetwork/1(in0)
  enb_counter_le_6/1 -> counter/Enable
  enb_counter_ge_8/1 -> enb_counter_ge_8_and_enb_counter_le_13/1
  in10/1 -> mux/6
  in4/1 -> mux/3
  in5/1 -> mux1/3
  in12/1 -> mux/7
  in2/1 -> mux/2
  in0/1 -> mux/1
  in1/1 -> mux1/1
  in6/1 -> mux/4
  enb_counter/1 -> enb_counter_le_6/1, enb_counter_ge_8/1, enb_counter_le_13/1, enb_counter_eq_14/1
  in8/1 -> mux/5
  in9/1 -> mux1/5
